simulink model "q4_a_simulink_PD"  (R2013a)
settings: Solver=ode45  StartTime=0.0  StopTime=100.0  RelTol=1e-3
values from neighbouring files (symbols this model uses):
  Kd = Kd_temp    [f.m]    (also in q4_a_PD.m = x1)
  Kp = Kp_temp    [f.m]    (also in q4_a_PD.m = x2)
settings Model: Creator=obrien94  LastModifiedBy=obrien94

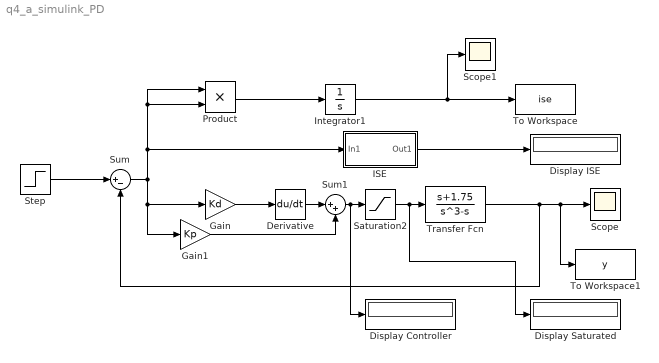
== system q4_a_simulink_PD ==
  Derivative : Derivative
  Display Controller : Display
  Display ISE : Display
  Display Saturated : Display
  Gain : Gain  Gain=Kd
  Gain1 : Gain  Gain=Kp
  ISE : Subsystem
      mask help:
      | ISE performance index
      |
      | output = int (input)^2 dt
      mask Display:
      | disp('ISE')
      | port_label('input',1,'e')
      | port_label('output',1,'ise')
  Integrator1 : Integrator
  Product : Product
  Saturation2 : Saturate  UpperLimit=5  LowerLimit=-5
  Scope : Scope
  Scope1 : Scope
  Step : Step  SampleTime=0
  Sum : Sum  Inputs=|+-
  Sum1 : Sum  Inputs=|++
  To Workspace : ToWorkspace  VariableName=ise  SampleTime=-1
  To Workspace1 : ToWorkspace  VariableName=y  SampleTime=-1  SaveFormat=Timeseries
  Transfer Fcn : TransferFcn  Numerator=[1 1.75]  Denominator=[1 0 -1 0]
  wires:
  Step/1 -> Sum/1
  Sum/1 -> Gain1/1, Gain/1, Product/1, Product/2, ISE/1(In1)
  Product/1 -> Integrator1/1
  Integrator1/1 -> Scope1/1, To Workspace/1
  Transfer Fcn/1 -> Sum/2, To Workspace1/1, Scope/1
  Derivative/1 -> Sum1/1
  ISE/1(Out1) -> Display ISE/1
  Sum1/1 -> Display Controller/1, Saturation2/1
  Gain/1 -> Derivative/1
  Gain1/1 -> Sum1/2
  Saturation2/1 -> Display Saturated/1, Transfer Fcn/1

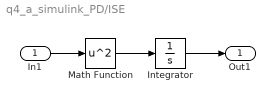
== system q4_a_simulink_PD/ISE ==
  In1 : Inport
  Integrator : Integrator
  Math Function : Math  Operator=square  SaturateOnIntegerOverflow=on
  Out1 : Outport
  wires:
  Math Function/1 -> Integrator/1
  Integrator/1 -> Out1/1
  In1/1 -> Math Function/1
